simulink model "motor_DC"  (R2018a)
settings: Solver=VariableStepAuto  StartTime=0.0  StopTime=0.04  RelTol=1e-3
values from neighbouring files (symbols this model uses):
  b = 0.1    [motord_DC_rot.m]
  J = 0.01    [motord_DC_rot.m]
  Kb = 5    [motord_DC_rot.m]
  Kp = 5    [motord_DC_rot.m]
  L = 1e-3    (= 0.001)    [motord_DC_rot.m]
  R = 10    [motord_DC_rot.m]
settings Model: Creator=carma  LastModifiedBy=carma

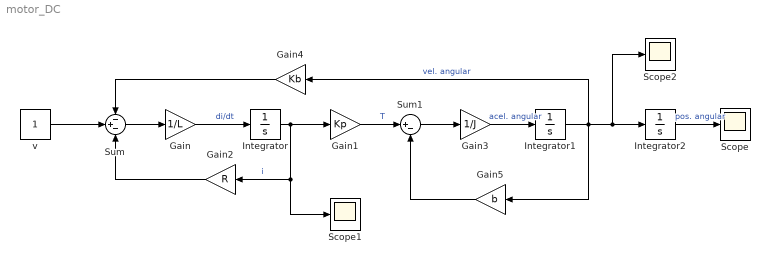
== system motor_DC ==
  Gain : Gain  Gain=1/L
  Gain1 : Gain  Gain=Kp
  Gain2 : Gain  Gain=R
  Gain3 : Gain  Gain=1/J
  Gain4 : Gain  Gain=Kb
  Gain5 : Gain  Gain=b
  Integrator : Integrator
  Integrator1 : Integrator
  Integrator2 : Integrator
  Scope : Scope
  Scope1 : Scope
  Scope2 : Scope
  Sum : Sum  Inputs=-+-
  Sum1 : Sum  Inputs=|+-
  v : Constant
  wires:
  v/1 -> Sum/2
  Sum/1 -> Gain/1
  Gain/1 -> Integrator/1  "di/dt"
  Integrator/1 -> Scope1/1, Gain2/1, Gain1/1  "i"
  Gain2/1 -> Sum/3
  Gain1/1 -> Sum1/1  "T"
  Sum1/1 -> Gain3/1
  Gain3/1 -> Integrator1/1  "acel. angular"
  Integrator1/1 -> Gain4/1, Gain5/1, Scope2/1, Integrator2/1  "vel. angular"
  Integrator2/1 -> Scope/1  "pos. angular"
  Gain5/1 -> Sum1/2
  Gain4/1 -> Sum/1
